simulink model "UAV_sync_unknown_sim"  (R2018b)
settings: Solver=ode23tb  StartTime=0.0  StopTime=35  RelTol=1e-3
values from neighbouring files (symbols this model uses):
  Bm = [zeros(6,6); eye(6)]    [UAV_sync_unknown.m]    (also in UAV_sync_unknown_gap.m)
  C_rho = 1.225    [SC42120_UAV_Preconditions.m]
  D0 = [M0 0 0 0 0 0 ... (first row only)    [SC42120_UAV_Preconditions.m]
  Derivative_gain_phi = 50    [SC42120_UAV_Preconditions.m]
  Derivative_gain_psi = 50    [SC42120_UAV_Preconditions.m]
  Derivative_gain_theta = 50    [SC42120_UAV_Preconditions.m]
  Derivative_gain_x = 50    [SC42120_UAV_Preconditions.m]
  Derivative_gain_y = 50    [SC42120_UAV_Preconditions.m]
  Derivative_gain_z = 50    [SC42120_UAV_Preconditions.m]
  G = 9.80665    [SC42120_UAV_Preconditions.m]
  g0 = [0;0;-M0*G;0;0;0]    [SC42120_UAV_Preconditions.m]
  I0 = [0.02 0 -0.01 ... (first row only)    [SC42120_UAV_Preconditions.m]
  InitWind = [0;0;0]    [SC42120_UAV_Preconditions.m]
  Kp = diag(P)    [SC42120_UAV_Preconditions.m]
  Kv = diag(V)    [SC42120_UAV_Preconditions.m]
  M0 = 10    [SC42120_UAV_Preconditions.m]
  M1 = 20    [UAV_sync_known.m]    (also in UAV_sync_unknown.m; UAV_sync_unknown_gap.m)
  M2 = 30    [UAV_sync_known.m]    (also in UAV_sync_unknown.m; UAV_sync_unknown_gap.m)
  M3 = 40    [UAV_sync_known.m]    (also in UAV_sync_unknown.m; UAV_sync_unknown_gap.m)
  M4 = 50    [UAV_sync_known.m]    (also in UAV_sync_unknown.m; UAV_sync_unknown_gap.m)
  P = [Proportional_x Proportional_y Proportional_z Proportional_phi Proportional_theta Proportional_psi]    [SC42120_UAV_Preconditions.m]    (also in UAV_sync_unknown.m = lyap(Am',Q); UAV_sync_unknown_gap.m = lyap(Am',Q); drawDATCOMaircraft.m = temparray)
  Proportional_phi = 50    [SC42120_UAV_Preconditions.m]
  Proportional_psi = 50    [SC42120_UAV_Preconditions.m]
  Proportional_theta = 50    [SC42120_UAV_Preconditions.m]
  Proportional_x = 50    [SC42120_UAV_Preconditions.m]
  Proportional_y = 50    [SC42120_UAV_Preconditions.m]
  Proportional_z = 50    [SC42120_UAV_Preconditions.m]
undefined symbols (not defined in the file or in its folder): Aero, APlane, Bxl, C, Ctr, deg, DiscIntNeverNeededParam, F, Guid, Init, Light, MIL, Path, rad, s, Trim, Utility
libraries: aerolibconvert2 x37, sharedutil x18, simulink x15, dspsigops x7, shared6dof x6, aerolibasang x4, simulink_extras x3, aerolibadyn x1, aerolibtransform2 x1, aerolibwind2 x1
(part 2 of 7)

== system UAV_sync_unknown_sim/Node 0/VF Approach/ENVIRONMENT ==
  note: Wind slowly time varying
  note: Dynamic wind
  note: Constant wind
  PlantData : Inport
  Bus Creator : BusCreator  Inputs=4
  Bus Selector1 : BusSelector  OutputSignals=xyh,Velocity (inertial),From inertial to body matrix
  Bus Selector2 : BusSelector  OutputSignals=From inertial to body matrix
  Bus Selector3 : BusSelector  OutputSignals=PlantData
  Bus Selector4 : BusSelector  OutputSignals=From inertial to body matrix
  Constant1 : Constant  Value=Init.windConst
  Dot Product : DotProduct  InputSameDT=on  OutDataTypeStr=Inherit: Inherit via internal rule
  Dryden Wind Turbulence Model (Continuous (+q +r)) : aerolibwind2/Dryden Wind Turbulence Model  (Continuous (+q -r))  units=Metric (MKS)  spec=MIL-F-8785C  model=Continuous Dryden (+q +r)  W20=10  Wdeg=135  TurbProb=10^-2 - Light  L_high=533.4  Wingspan=Bxl.b  ts=0.1  Seed=[23341 23342 23343 23344]  T_on=on
      settings: SourceProductName=Aerospace Blockset
  Height : Selector  InputPortWidth=3  IndexOptions=Index vector (dialog)  Indices=3  OutputSizes=1
  Init.DryOnOff : Gain  Gain=Init.DryOnOff
  "Init.DryOnOff " : Gain  Gain=Init.DryOnOff
  Init.WTimevar : Gain  Gain=Init.WTimevar
  Product : Product  Multiplication=Matrix(*)
  "Product " : Product  Multiplication=Matrix(*)
  Slowly time varying wind gen. : Subsystem
  Sum1 : Sum  Inputs=|++
  Sum3 : Sum  Inputs=|++
  Vt : Sqrt  SaturateOnIntegerOverflow=on
  EnvData : Outport
  wires:
  Bus Selector1/1 -> Height/1  "<xyh>"
  Bus Selector1/2 -> Dot Product/2, Dot Product/1  "<Velocity (inertial)>"
  Bus Selector1/3 -> Dryden Wind Turbulence Model (Continuous (+q +r))/3  "<From inertial to body matrix>"
  Bus Selector3/1 -> Bus Selector4/1, Bus Selector1/1, Bus Selector2/1  "<PlantData>"
  Height/1 -> Dryden Wind Turbulence Model (Continuous (+q +r))/1  "Altitude"
  Dot Product/1 -> Vt/1
  Vt/1 -> Dryden Wind Turbulence Model (Continuous (+q +r))/2  "Speed"
  Sum1/1 -> Bus Creator/3, Sum3/2  "Wind velocity (dyn) (body)"
  Constant1/1 -> Product/2
  Bus Creator/1 -> EnvData/1
  "Init.DryOnOff "/1 -> Bus Creator/4  "Wind ang rate (dyn) (body)"
  Sum3/1 -> Bus Creator/2  "Wind total (body)"
  Dryden Wind Turbulence Model (Continuous (+q +r))/1 -> Init.DryOnOff/1
  Bus Selector2/1 -> Product/1  "<From inertial to body matrix>"
  Dryden Wind Turbulence Model (Continuous (+q +r))/2 -> "Init.DryOnOff "/1
  PlantData/1 -> Bus Selector3/1
  Product/1 -> Bus Creator/1, Sum3/1  "Wind velocity (sta) (body)"
  Bus Selector4/1 -> "Product "/1  "<From inertial to body matrix>"
  Init.WTimevar/1 -> Sum1/2  "Wind slowly time varying"
  Init.DryOnOff/1 -> Sum1/1
  "Product "/1 -> Init.WTimevar/1
  Slowly time varying wind gen./1(Out1) -> "Product "/2

== system UAV_sync_unknown_sim/Node 0/VF Approach/GROUND HIT ==
  PlantData : Inport
  Bus Selector1 : BusSelector  OutputSignals=xyh
  Bus Selector3 : BusSelector  OutputSignals=PlantData
  Constant : Constant  Value=0
  Relational Operator : RelationalOperator  Operator=<=  OutDataTypeStr=boolean  RndMeth=Simplest
  Selector : Selector  InputPortWidth=3  IndexOptions=Index vector (dialog)  Indices=3  OutputSizes=1
  Stop Simulation : Stop
  wires:
  PlantData/1 -> Bus Selector3/1
  Selector/1 -> Relational Operator/1
  Bus Selector1/1 -> Selector/1  "<xyh>"
  Constant/1 -> Relational Operator/2
  Relational Operator/1 -> Stop Simulation/1
  Bus Selector3/1 -> Bus Selector1/1  "<PlantData>"

== system UAV_sync_unknown_sim/Node 0/VF Approach/MANUAL INPUTS ==
  note: Manual control
      |
      | The switches below enable (up position) or disable (down position) the manual control in the Visual Interface sub-block.
      | (default: down)
  note: Open-loop inputs
      |
      | The switches below enables a custom input from the Workspace (timeseries data type) to the control surfaces.
  note: Trim condition
      |
      | The sub-block below allows to try the actuators configuration for a trimmed flight.
  CtrBus : Inport
  EnvData : Inport  Port=2
  VF : Inport  Port=3
  GuidData : Inport  Port=4
  Bus Creator : BusCreator  Inputs=7
  Bus Selector : BusSelector  OutputSignals=throttle,ailerons,elevator,rudder
  Bus Selector1 : BusSelector  OutputSignals=Out_references,Target_height,Target_airspeed
  "CtrBus " : InportShadow
  From Workspace1 : FromWorkspace  Commented=on  VariableName=LogData.RCIN.ElevDem_IN  SampleTime=0.001
  From Workspace2 : FromWorkspace  Commented=on  VariableName=LogData.RCIN.RuddDem_IN  SampleTime=0.001
  From Workspace3 : FromWorkspace  Commented=on  VariableName=LogData.RCIN.ThrottleDem_IN  SampleTime=0.001
  From Workspace4 : FromWorkspace  Commented=on  VariableName=LogData.RCIN.AilDem_IN  SampleTime=0.001
  Goto4 : Goto  Commented=on  GotoTag=throttle
  Manual Switch{,1..7} (8 alike) : ManualSwitch  CurrentSetting=0
  Manual_cmd{,4..6} (4 alike) : Constant  Value=0
  Trim conditions : Subsystem
  CtrBus. : Outport
  EnvData. : Outport  Port=2
  GuidData. : Outport  Port=3
  VF. : Outport  Port=4
  wires:
  Manual Switch4/1 -> Goto4/1, Bus Creator/1  "throttle"
  Manual Switch7/1 -> Bus Creator/3  "elevator"
  Manual_cmd/1 -> Manual Switch/1
  Manual_cmd4/1 -> Manual Switch1/1
  Manual Switch5/1 -> Bus Creator/2  "ailerons"
  Manual Switch6/1 -> Bus Creator/4  "rudder"
  Manual_cmd6/1 -> Manual Switch3/1
  Manual_cmd5/1 -> Manual Switch2/1
  Bus Creator/1 -> CtrBus./1
  Manual Switch1/1 -> Manual Switch5/2  "ailerons"
  Manual Switch2/1 -> Manual Switch7/2  "elevator"
  Manual Switch3/1 -> Manual Switch6/2  "rudder"
  From Workspace3/1 -> Manual Switch4/1
  Manual Switch/1 -> Manual Switch4/2
  Bus Selector/1 -> Trim conditions/1(throttle)  "<throttle>"
  Trim conditions/1(throttout) -> Manual Switch/2
  Bus Selector/2 -> Trim conditions/2(ail)  "<ailerons>"
  Bus Selector/3 -> Trim conditions/3(elev)  "<elevator>"
  Bus Selector/4 -> Trim conditions/4(rudd)  "<rudder>"
  Trim conditions/4(ruddout) -> Manual Switch3/2
  Trim conditions/2(ailout) -> Manual Switch1/2
  Trim conditions/3(elevout) -> Manual Switch2/2
  EnvData/1 -> EnvData./1
  From Workspace4/1 -> Manual Switch5/1
  From Workspace1/1 -> Manual Switch7/1
  From Workspace2/1 -> Manual Switch6/1
  GuidData/1 -> GuidData./1
  VF/1 -> VF./1
  CtrBus/1 -> Bus Selector/1
  "CtrBus "/1 -> Bus Selector1/1
  Bus Selector1/1 -> Bus Creator/5  "<Out_references>"
  Bus Selector1/2 -> Bus Creator/6  "<Target_height>"
  Bus Selector1/3 -> Bus Creator/7  "<Target_airspeed>"

== system UAV_sync_unknown_sim/Node 0/VF Approach/PATH FOLLOWING ==
  note: Out
  note: Ground speed(s) calculation
  note: Output merge
  note: Path following
      |
      | Each subsystem is enabled by the 'flag' variable according to the path manager choice or user configuration.
      | If you want to use only the path following for a single line/orbit simulation, then disable the Path manager.
      |
      | GPS-derived signals, such as the inertial position and the course angle use a 10 Hz sampling time to reflect real signal on-board acquisition.
  PlantData : Inport
  DerCond : Inport  Port=2
  EnvData : Inport  Port=3
  GuidData : Inport  Port=4
  Angle Conversion : aerolibconvert2/Angle Conversion  IU=rad  OU=deg
  Bus Creator : BusCreator  Inputs=7
  Bus Selector{1,4,6,8} (4 alike) : BusSelector  OutputSignals=PlantData
  Bus Selector2 : BusSelector  OutputSignals=DerCond
  Bus Selector3 : BusSelector  OutputSignals=DerCond
  Bus Selector5 : BusSelector  OutputSignals=Path flag
  Constant6 : Constant  Value=0
  Data Type Conversion : DataTypeConversion  OutDataTypeStr=boolean
  "DerCond " : InportShadow  Port=2
  "EnvData " : InportShadow  Port=3
  Extract Vg : Subsystem
  Extract Vg_prime : Subsystem
  "GuidData " : InportShadow  Port=4
  Logical Operator : Logic  Operator=NOT  AllPortsSameDT=off  OutDataTypeStr=boolean
  Manual Switch1 : ManualSwitch  CurrentSetting=0
  Merge{,1..3} (4 alike) : Merge
  Orbit Path Following (Enabled Subsystem) : Subsystem  TreatAsAtomicUnit=on
  "PlantData " : InportShadow
  "PlantData  " : InportShadow
  "PlantData   " : InportShadow
  Scope : Scope
  Straight-line Path Following (Enabled Subsystem) : Subsystem  TreatAsAtomicUnit=on
  "PlantData. " : Outport
  "DerCond. " : Outport  Port=2
  EnvData. : Outport  Port=3
  VF. : Outport  Port=4
  GuidData. : Outport  Port=5
  wires:
  Merge/1 -> Manual Switch1/2
  Constant6/1 -> Manual Switch1/1
  EnvData/1 -> EnvData./1
  PlantData/1 -> Bus Selector4/1, Bus Selector1/1
  Bus Selector1/1 -> Straight-line Path Following (Enabled Subsystem)/1(PlantData)  "<PlantData>"
  DerCond/1 -> Bus Selector2/1, Bus Selector3/1
  Bus Creator/1 -> VF./1
  Manual Switch1/1 -> Bus Creator/2, Angle Conversion/1  "chi_c"
  Logical Operator/1 -> Orbit Path Following (Enabled Subsystem)/Enable
  Bus Selector4/1 -> Orbit Path Following (Enabled Subsystem)/1(PlantData)  "<PlantData>"
  Bus Selector3/1 -> Orbit Path Following (Enabled Subsystem)/2(DerCond)  "<DerCond>"
  Data Type Conversion/1 -> [path_flag], Straight-line Path Following (Enabled Subsystem)/Enable
  [path_flag] -> Logical Operator/1
  Bus Selector2/1 -> Straight-line Path Following (Enabled Subsystem)/2(DerCond)  "<DerCond>"
  Merge1/1 -> Bus Creator/3, Scope/1  "Vg_hat"
  [Vg_prime] -> Bus Creator/4  "Vg_prime"
  Straight-line Path Following (Enabled Subsystem)/2(Vg_hat_SL) -> [Vg_hat_SL]
  Straight-line Path Following (Enabled Subsystem)/3(chi_d_SL) -> [chi_d_SL]
  Straight-line Path Following (Enabled Subsystem)/4(chi_c_SL) -> [chi_c_SL]
  Orbit Path Following (Enabled Subsystem)/2(Vg_hat_O) -> [Vg_hat_O]
  Orbit Path Following (Enabled Subsystem)/3(chi_d_O) -> [chi_d_O]
  Orbit Path Following (Enabled Subsystem)/1(chi_c_O) -> [chi_c_O]
  [chi_c_SL] -> Merge/1
  [chi_c_O] -> Merge/2
  [Vg_hat_O] -> Merge1/2
  [Vg_hat_SL] -> Merge1/1
  [chi_d_O] -> Merge2/2
  [chi_d_SL] -> Merge2/1
  Merge2/1 -> Bus Creator/6  "chi_d"
  Angle Conversion/1 -> Bus Creator/1  "chi_c_deg"
  Straight-line Path Following (Enabled Subsystem)/1(e_y) -> [e_y]
  [e_y] -> Merge3/1
  Orbit Path Following (Enabled Subsystem)/4(d_tilde) -> [d_tilde]
  [d_tilde] -> Merge3/2
  Merge3/1 -> Bus Creator/7  "xtrack_erorr"
  GuidData/1 -> Bus Selector5/1, Orbit Path Following (Enabled Subsystem)/3(GuidData), Straight-line Path Following (Enabled Subsystem)/3(GuidData)
  Bus Selector5/1 -> Data Type Conversion/1  "<Path flag>"
  "DerCond "/1 -> "DerCond. "/1
  "GuidData "/1 -> GuidData./1
  "PlantData "/1 -> "PlantData. "/1
  Extract Vg_prime/1(Vg') -> [Vg_prime]
  Bus Selector6/1 -> Extract Vg_prime/1(PlantData)  "<PlantData>"
  [V_g] -> Bus Creator/5  "V_g"
  Extract Vg/1(Vg) -> [V_g]
  "PlantData  "/1 -> Bus Selector6/1
  [V_g] -> Straight-line Path Following (Enabled Subsystem)/4(Vg)
  [V_g] -> Orbit Path Following (Enabled Subsystem)/4(Vg)
  [Vg_prime] -> Straight-line Path Following (Enabled Subsystem)/5(Vg_prime)
  [Vg_prime] -> Orbit Path Following (Enabled Subsystem)/5(Vg_prime)
  "EnvData "/1 -> Extract Vg/2(EnvData)
  "PlantData   "/1 -> Bus Selector8/1
  Bus Selector8/1 -> Extract Vg/1(PlantData)  "<PlantData>"

== system UAV_sync_unknown_sim/Node 0/VF Approach/PATH MANAGER ==
  note: Path following only
  note: Path manager
  PlantData : Inport
  DerCond : Inport  Port=2
  EnvData : Inport  Port=3
  Bus Selector : BusSelector  OutputSignals=PlantData.Position (inertial)
  Constant : Constant  Value=Path.onOff
  Constant1 : Constant  Value=Path.onOff
  Data Type Conversion : DataTypeConversion  OutDataTypeStr=boolean
  Enabled Subsystem : Subsystem  TreatAsAtomicUnit=on
  Fcn : Fcn  Commented=on  Expr=u(1)
  Fcn1 : Fcn  Commented=on  Expr=u(2)
  Logical Operator : Logic  Operator=NOT  AllPortsSameDT=off  OutDataTypeStr=boolean
  Merge : Merge
  Path Following data : Subsystem  TreatAsAtomicUnit=on
  XY Graph : simulink/Sinks/XY Graph  Commented=on  xmin=-50  xmax=600  ymin=-50  ymax=600  st=0.1
  Plantdata. : Outport
  DerCond. : Outport  Port=2
  EnvData. : Outport  Port=3
  GuidData. : Outport  Port=4
  wires:
  PlantData/1 -> Bus Selector/1, Plantdata./1
  DerCond/1 -> DerCond./1
  EnvData/1 -> EnvData./1
  Bus Selector/1 -> Fcn1/1, Fcn/1, Enabled Subsystem/1(xy)  "<Position (inertial)>"
  Merge/1 -> GuidData./1
  Constant/1 -> Data Type Conversion/1
  Data Type Conversion/1 -> Enabled Subsystem/Enable
  Constant1/1 -> Logical Operator/1
  Logical Operator/1 -> Path Following data/Enable
  Enabled Subsystem/1(GuidData) -> Merge/1
  Path Following data/1(GuidData) -> Merge/2
  Fcn/1 -> XY Graph/1
  Fcn1/1 -> XY Graph/2

== system UAV_sync_unknown_sim/Node 0/VF Approach/TO WORKSPACE ==
  PlantData : Inport
  DerCond : Inport  Port=2
  ControlBus : Inport  Port=3
  VF : Inport  Port=4
  GuidData : Inport  Port=5
  EnvData : Inport  Port=6
  Bus Creator : BusCreator  Inputs=6
  Bus Selector4 : BusSelector  OutputSignals=DerCond
  Bus Selector5 : BusSelector  OutputSignals=PlantData
  Sample at 0.01s : ZeroOrderHold  SampleTime=0.01
  To Workspace2 : ToWorkspace  VariableName=SimOut  SaveFormat=Timeseries  SampleTime=-1
      settings: Save2DSignal=2-D array (concatenate along first dimension)
  wires:
  Bus Creator/1 -> Sample at 0.01s/1
  Bus Selector5/1 -> Bus Creator/1  "<PlantData>"
  PlantData/1 -> Bus Selector5/1
  ControlBus/1 -> Bus Creator/3  "ControlBus"
  DerCond/1 -> Bus Selector4/1
  Bus Selector4/1 -> Bus Creator/2  "<DerCond>"
  GuidData/1 -> Bus Creator/5  "GuidData"
  VF/1 -> Bus Creator/4  "VF"
  EnvData/1 -> Bus Creator/6  "EnvData"
  Sample at 0.01s/1 -> To Workspace2/1

== system UAV_sync_unknown_sim/Node 1/Node 1/eps_c1_transpose ==
  euler angles : Inport
  Constant : Constant  Value=zeros(3)
  Constant1 : Constant  Value=zeros(6,1)
  Constant{2..3,6..7} (4 alike) : Constant  Value=0
  Constant4 : Constant  Value=zeros(3)
  Constant5 : Constant  Value=zeros(6,1)
  Constant8 : Constant  Value=zeros(3)
  Constant9 : Constant  Value=zeros(6,1)
  Create 3x3 Matrix{,1..3} (4 alike) : sharedutil/Create 3x3 Matrix  aMode=aMode
  Demux : Demux  Outputs=3
  Gain{,1..7} (8 alike) : Gain  Gain=-1
  Matrix Concatenate{,2,5..6} (4 alike) : Concatenate  Mode=Multidimensional array
  Matrix Concatenate{1,3..4,7..9} (6 alike) : Concatenate  Mode=Multidimensional array  ConcatenateDimension=2
  eps_c : Outport
  wires:
  euler angles/1 -> Demux/1
  Demux/1 -> Gain6/1, Create 3x3 Matrix3/2, Gain/1, Create 3x3 Matrix/6, Create 3x3 Matrix1/7, Gain3/1  "p"
  Gain/1 -> Create 3x3 Matrix/8
  Demux/2 -> Create 3x3 Matrix2/1, Gain4/1, Create 3x3 Matrix/7, Gain1/1  "q"
  Gain1/1 -> Create 3x3 Matrix/3
  Demux/3 -> Gain7/1, Create 3x3 Matrix3/6, Create 3x3 Matrix2/5, Gain5/1, Gain2/1, Create 3x3 Matrix/2  "r"
  Gain2/1 -> Create 3x3 Matrix/4
  Create 3x3 Matrix/1 -> Matrix Concatenate/1
  Constant/1 -> Matrix Concatenate/2
  Matrix Concatenate/1 -> Matrix Concatenate1/1
  Constant1/1 -> Matrix Concatenate1/2
  Constant2/1 -> Create 3x3 Matrix/9, Create 3x3 Matrix/5, Create 3x3 Matrix/1
  Constant3/1 -> Create 3x3 Matrix1/8, Create 3x3 Matrix1/6, Create 3x3 Matrix1/4, Create 3x3 Matrix1/3, Create 3x3 Matrix1/2, Create 3x3 Matrix1/1
  Gain3/1 -> Create 3x3 Matrix1/5
  Gain4/1 -> Create 3x3 Matrix1/9
  Create 3x3 Matrix1/1 -> Matrix Concatenate2/2
  Constant4/1 -> Matrix Concatenate2/1
  Matrix Concatenate1/1 -> Matrix Concatenate3/1
  Matrix Concatenate2/1 -> Matrix Concatenate3/2
  Matrix Concatenate3/1 -> Matrix Concatenate4/1
  Constant5/1 -> Matrix Concatenate4/2
  Gain5/1 -> Create 3x3 Matrix2/3
  Constant6/1 -> Create 3x3 Matrix2/9, Create 3x3 Matrix2/8, Create 3x3 Matrix2/7, Create 3x3 Matrix2/6, Create 3x3 Matrix2/4, Create 3x3 Matrix2/2
  Gain6/1 -> Create 3x3 Matrix3/4
  Gain7/1 -> Create 3x3 Matrix3/8
  Constant7/1 -> Create 3x3 Matrix3/9, Create 3x3 Matrix3/7, Create 3x3 Matrix3/5, Create 3x3 Matrix3/3, Create 3x3 Matrix3/1
  Create 3x3 Matrix2/1 -> Matrix Concatenate5/2
  Constant8/1 -> Matrix Concatenate6/1, Matrix Concatenate5/1
  Create 3x3 Matrix3/1 -> Matrix Concatenate6/2
  Constant9/1 -> Matrix Concatenate7/2
  Matrix Concatenate5/1 -> Matrix Concatenate7/1
  Matrix Concatenate7/1 -> Matrix Concatenate8/1
  Matrix Concatenate6/1 -> Matrix Concatenate8/2
  Matrix Concatenate4/1 -> Matrix Concatenate9/1
  Matrix Concatenate8/1 -> Matrix Concatenate9/2
  Matrix Concatenate9/1 -> eps_c/1

== system UAV_sync_unknown_sim/Node 1/Node 1/eps_g ==
  euler angles : Inport
  Cos : Trigonometry  Operator=cos
  Cos1 : Trigonometry  Operator=cos
  Demux : Demux  Outputs=3
  Gain : Gain  Gain=G
  Gain1 : Gain  Gain=G
  Gain2 : Gain  Gain=G
  Gain3 : Gain  Gain=-1
  Gain4 : Gain  Gain=-1
  Multiply : Product
  Multiply1 : Product
  Mux : Mux  Inputs=6
  Sin : Trigonometry
  Sin1 : Trigonometry
  Sin2 : Trigonometry  Operator=cos
  Terminator : Terminator
  Zero : Constant  Value=0  OutDataTypeStr=Inherit: Inherit via back propagation
  eps_g : Outport
  wires:
  euler angles/1 -> Demux/1
  Sin/1 -> Gain/1
  Cos/1 -> Multiply/1
  Sin1/1 -> Multiply/2
  Multiply/1 -> Gain1/1
  Cos1/1 -> Multiply1/1
  Sin2/1 -> Multiply1/2
  Multiply1/1 -> Gain2/1
  Gain/1 -> Mux/1
  Gain1/1 -> Gain3/1
  Gain2/1 -> Gain4/1
  Zero/1 -> Mux/6, Mux/4, Mux/5
  Mux/1 -> eps_g/1
  Gain3/1 -> Mux/2
  Gain4/1 -> Mux/3
  Demux/1 -> Cos1/1, Sin1/1
  Demux/2 -> Sin2/1, Cos/1, Sin/1
  Demux/3 -> Terminator/1

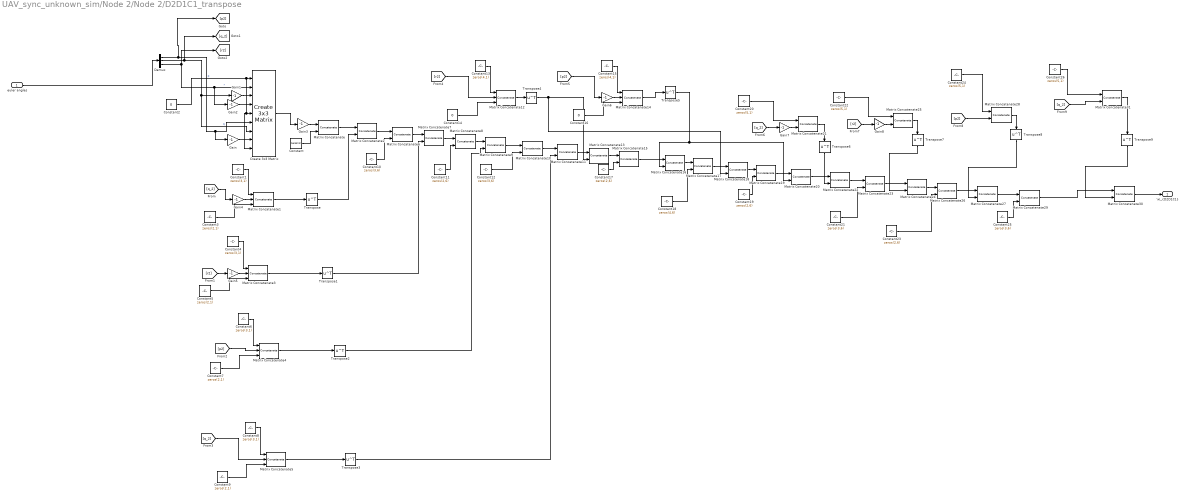
== system UAV_sync_unknown_sim/Node 2/Node 2/D2D1C1_transpose ==
  euler angles : Inport
  Constant : Constant  Value=zeros(3)
  Constant{1,4,6,8} (4 alike) : Constant  Value=zeros(3,1)
  Constant{10,12,21,25} (4 alike) : Constant  Value=zeros(3,6)
  Constant{11,17,19,23} (4 alike) : Constant  Value=zeros(2,6)
  Constant13 : Constant  Value=zeros(4,1)
  Constant14 : Constant  Value=0
  Constant15 : Constant  Value=zeros(4,1)
  Constant16 : Constant  Value=0
  Constant18 : Constant  Value=zeros(4,6)
  Constant2 : Constant  Value=0
  Constant{20,22,24,26} (4 alike) : Constant  Value=zeros(5,1)
  Constant{3,5,7,9} (4 alike) : Constant  Value=zeros(2,1)
  Create 3x3 Matrix : sharedutil/Create 3x3 Matrix  aMode=aMode
  Demux : Demux  Outputs=3
  Gain{,1..8} (9 alike) : Gain  Gain=-1
  Matrix Concatenate : Concatenate  Mode=Multidimensional array  ConcatenateDimension=2
  Matrix Concatenate{1,3..5,12,14} (6 alike) : Concatenate  NumInputs=3  Mode=Multidimensional array
  Matrix Concatenate{2,6..11,13,15..31} (25 alike) : Concatenate  Mode=Multidimensional array
  Transpose{,1..9} (10 alike) : Math  Operator=transpose  SaturateOnIntegerOverflow=on
  "\\xi_{D2D1C1}" : Outport
  wires:
  euler angles/1 -> Demux/1
  Demux/1 -> [p2], Gain/1, Create 3x3 Matrix/6  "p"
  Gain/1 -> Create 3x3 Matrix/8
  Demux/2 -> [q_2], Create 3x3 Matrix/7, Gain1/1  "q"
  Gain1/1 -> Create 3x3 Matrix/3
  Demux/3 -> Gain2/1, Create 3x3 Matrix/2, [r2]  "r"
  Gain2/1 -> Create 3x3 Matrix/4
  Create 3x3 Matrix/1 -> Gain3/1
  Constant/1 -> Matrix Concatenate/2
  Matrix Concatenate/1 -> Matrix Concatenate2/1
  Constant2/1 -> Create 3x3 Matrix/9, Create 3x3 Matrix/5, Create 3x3 Matrix/1
  Gain3/1 -> Matrix Concatenate/1
  Constant1/1 -> Matrix Concatenate1/1
  Constant3/1 -> Matrix Concatenate1/3
  Gain4/1 -> Matrix Concatenate1/2
  Matrix Concatenate1/1 -> Transpose/1
  Gain5/1 -> Matrix Concatenate3/2
  Constant5/1 -> Matrix Concatenate3/3
  Constant4/1 -> Matrix Concatenate3/1
  Constant7/1 -> Matrix Concatenate4/3
  Constant6/1 -> Matrix Concatenate4/1
  Constant9/1 -> Matrix Concatenate5/3
  Constant8/1 -> Matrix Concatenate5/1
  [q_2] -> Gain4/1
  [r2] -> Gain5/1
  [p2] -> Matrix Concatenate4/2
  [q_2] -> Matrix Concatenate5/2
  Matrix Concatenate2/1 -> Matrix Concatenate6/1
  Constant10/1 -> Matrix Concatenate6/2
  Matrix Concatenate6/1 -> Matrix Concatenate7/1
  Matrix Concatenate3/1 -> Transpose1/1
  Matrix Concatenate7/1 -> Matrix Concatenate8/1
  Matrix Concatenate8/1 -> Matrix Concatenate9/1
  Constant11/1 -> Matrix Concatenate8/2
  Matrix Concatenate4/1 -> Transpose2/1
  Matrix Concatenate9/1 -> Matrix Concatenate10/1
  Constant12/1 -> Matrix Concatenate10/2
  Matrix Concatenate10/1 -> Matrix Concatenate11/1
  Matrix Concatenate5/1 -> Transpose3/1
  Constant13/1 -> Matrix Concatenate12/1
  Constant14/1 -> Matrix Concatenate12/3
  [r2] -> Matrix Concatenate12/2
  Matrix Concatenate12/1 -> Transpose4/1
  Matrix Concatenate11/1 -> Matrix Concatenate13/1
  Constant16/1 -> Matrix Concatenate14/3
  [p2] -> Gain6/1
  Constant15/1 -> Matrix Concatenate14/1
  Gain6/1 -> Matrix Concatenate14/2
  Matrix Concatenate13/1 -> Matrix Concatenate15/1
  Constant17/1 -> Matrix Concatenate15/2
  Matrix Concatenate15/1 -> Matrix Concatenate16/1
  Matrix Concatenate14/1 -> Transpose5/1
  Matrix Concatenate16/1 -> Matrix Concatenate17/1
  Constant18/1 -> Matrix Concatenate17/2
  Matrix Concatenate17/1 -> Matrix Concatenate18/1
  Matrix Concatenate18/1 -> Matrix Concatenate19/1
  Constant19/1 -> Matrix Concatenate19/2
  Matrix Concatenate19/1 -> Matrix Concatenate20/1
  Constant20/1 -> Matrix Concatenate21/1
  Gain7/1 -> Matrix Concatenate21/2
  [q_2] -> Gain7/1
  Matrix Concatenate21/1 -> Transpose6/1
  Matrix Concatenate20/1 -> Matrix Concatenate22/1
  Matrix Concatenate22/1 -> Matrix Concatenate23/1
  Constant21/1 -> Matrix Concatenate23/2
  Matrix Concatenate23/1 -> Matrix Concatenate24/1
  Gain8/1 -> Matrix Concatenate25/2
  Constant22/1 -> Matrix Concatenate25/1
  [r2] -> Gain8/1
  Matrix Concatenate25/1 -> Transpose7/1
  Matrix Concatenate24/1 -> Matrix Concatenate26/1
  Constant23/1 -> Matrix Concatenate26/2
  Matrix Concatenate26/1 -> Matrix Concatenate27/1
  Matrix Concatenate28/1 -> Transpose8/1
  [p2] -> Matrix Concatenate28/2
  Constant24/1 -> Matrix Concatenate28/1
  Matrix Concatenate27/1 -> Matrix Concatenate29/1
  Constant25/1 -> Matrix Concatenate29/2
  Matrix Concatenate29/1 -> Matrix Concatenate30/1
  Constant26/1 -> Matrix Concatenate31/1
  [q_2] -> Matrix Concatenate31/2
  Matrix Concatenate31/1 -> Transpose9/1
  Matrix Concatenate30/1 -> "\\xi_{D2D1C1}"/1
  Transpose/1 -> Matrix Concatenate2/2
  Transpose1/1 -> Matrix Concatenate7/2
  Transpose2/1 -> Matrix Concatenate9/2
  Transpose3/1 -> Matrix Concatenate11/2
  Transpose4/1 -> Matrix Concatenate18/2, Matrix Concatenate13/2
  Transpose5/1 -> Matrix Concatenate16/2, Matrix Concatenate20/2
  Transpose6/1 -> Matrix Concatenate22/2
  Transpose7/1 -> Matrix Concatenate24/2
  Transpose8/1 -> Matrix Concatenate27/2
  Transpose9/1 -> Matrix Concatenate30/2

== system UAV_sync_unknown_sim/Node 2/Node 2/eps_c1_transpose ==
  euler angles : Inport
  Constant : Constant  Value=zeros(3)
  Constant1 : Constant  Value=zeros(6,1)
  Constant{2..3,6..7} (4 alike) : Constant  Value=0
  Constant4 : Constant  Value=zeros(3)
  Constant5 : Constant  Value=zeros(6,1)
  Constant8 : Constant  Value=zeros(3)
  Constant9 : Constant  Value=zeros(6,1)
  Create 3x3 Matrix{,1..3} (4 alike) : sharedutil/Create 3x3 Matrix  aMode=aMode
  Demux : Demux  Outputs=3
  Gain{,1..7} (8 alike) : Gain  Gain=-1
  Matrix Concatenate{,2,5..6} (4 alike) : Concatenate  Mode=Multidimensional array
  Matrix Concatenate{1,3..4,7..9} (6 alike) : Concatenate  Mode=Multidimensional array  ConcatenateDimension=2
  eps_c : Outport
  wires:
  euler angles/1 -> Demux/1
  Demux/1 -> Gain6/1, Create 3x3 Matrix3/2, Gain/1, Create 3x3 Matrix/6, Create 3x3 Matrix1/7, Gain3/1  "p"
  Gain/1 -> Create 3x3 Matrix/8
  Demux/2 -> Create 3x3 Matrix2/1, Gain4/1, Create 3x3 Matrix/7, Gain1/1  "q"
  Gain1/1 -> Create 3x3 Matrix/3
  Demux/3 -> Gain7/1, Create 3x3 Matrix3/6, Create 3x3 Matrix2/5, Gain5/1, Gain2/1, Create 3x3 Matrix/2  "r"
  Gain2/1 -> Create 3x3 Matrix/4
  Create 3x3 Matrix/1 -> Matrix Concatenate/1
  Constant/1 -> Matrix Concatenate/2
  Matrix Concatenate/1 -> Matrix Concatenate1/1
  Constant1/1 -> Matrix Concatenate1/2
  Constant2/1 -> Create 3x3 Matrix/9, Create 3x3 Matrix/5, Create 3x3 Matrix/1
  Constant3/1 -> Create 3x3 Matrix1/8, Create 3x3 Matrix1/6, Create 3x3 Matrix1/4, Create 3x3 Matrix1/3, Create 3x3 Matrix1/2, Create 3x3 Matrix1/1
  Gain3/1 -> Create 3x3 Matrix1/5
  Gain4/1 -> Create 3x3 Matrix1/9
  Create 3x3 Matrix1/1 -> Matrix Concatenate2/2
  Constant4/1 -> Matrix Concatenate2/1
  Matrix Concatenate1/1 -> Matrix Concatenate3/1
  Matrix Concatenate2/1 -> Matrix Concatenate3/2
  Matrix Concatenate3/1 -> Matrix Concatenate4/1
  Constant5/1 -> Matrix Concatenate4/2
  Gain5/1 -> Create 3x3 Matrix2/3
  Constant6/1 -> Create 3x3 Matrix2/9, Create 3x3 Matrix2/8, Create 3x3 Matrix2/7, Create 3x3 Matrix2/6, Create 3x3 Matrix2/4, Create 3x3 Matrix2/2
  Gain6/1 -> Create 3x3 Matrix3/4
  Gain7/1 -> Create 3x3 Matrix3/8
  Constant7/1 -> Create 3x3 Matrix3/9, Create 3x3 Matrix3/7, Create 3x3 Matrix3/5, Create 3x3 Matrix3/3, Create 3x3 Matrix3/1
  Create 3x3 Matrix2/1 -> Matrix Concatenate5/2
  Constant8/1 -> Matrix Concatenate6/1, Matrix Concatenate5/1
  Create 3x3 Matrix3/1 -> Matrix Concatenate6/2
  Constant9/1 -> Matrix Concatenate7/2
  Matrix Concatenate5/1 -> Matrix Concatenate7/1
  Matrix Concatenate7/1 -> Matrix Concatenate8/1
  Matrix Concatenate6/1 -> Matrix Concatenate8/2
  Matrix Concatenate4/1 -> Matrix Concatenate9/1
  Matrix Concatenate8/1 -> Matrix Concatenate9/2
  Matrix Concatenate9/1 -> eps_c/1

== system UAV_sync_unknown_sim/Node 2/Node 2/eps_g ==
  euler angles : Inport
  Cos : Trigonometry  Operator=cos
  Cos1 : Trigonometry  Operator=cos
  Demux : Demux  Outputs=3
  Gain : Gain  Gain=G
  Gain1 : Gain  Gain=G
  Gain2 : Gain  Gain=G
  Gain3 : Gain  Gain=-1
  Gain4 : Gain  Gain=-1
  Multiply : Product
  Multiply1 : Product
  Mux : Mux  Inputs=6
  Sin : Trigonometry
  Sin1 : Trigonometry
  Sin2 : Trigonometry  Operator=cos
  Terminator : Terminator
  Zero : Constant  Value=0  OutDataTypeStr=Inherit: Inherit via back propagation
  eps_g : Outport
  wires:
  euler angles/1 -> Demux/1
  Sin/1 -> Gain/1
  Cos/1 -> Multiply/1
  Sin1/1 -> Multiply/2
  Multiply/1 -> Gain1/1
  Cos1/1 -> Multiply1/1
  Sin2/1 -> Multiply1/2
  Multiply1/1 -> Gain2/1
  Gain/1 -> Mux/1
  Gain1/1 -> Gain3/1
  Gain2/1 -> Gain4/1
  Zero/1 -> Mux/6, Mux/4, Mux/5
  Mux/1 -> eps_g/1
  Gain3/1 -> Mux/2
  Gain4/1 -> Mux/3
  Demux/1 -> Cos1/1, Sin1/1
  Demux/2 -> Sin2/1, Cos/1, Sin/1
  Demux/3 -> Terminator/1

== system UAV_sync_unknown_sim/Node 3/Node 1/eps_c1_transpose ==
  euler angles : Inport
  Constant : Constant  Value=zeros(3)
  Constant1 : Constant  Value=zeros(6,1)
  Constant{2..3,6..7} (4 alike) : Constant  Value=0
  Constant4 : Constant  Value=zeros(3)
  Constant5 : Constant  Value=zeros(6,1)
  Constant8 : Constant  Value=zeros(3)
  Constant9 : Constant  Value=zeros(6,1)
  Create 3x3 Matrix{,1..3} (4 alike) : sharedutil/Create 3x3 Matrix  aMode=aMode
  Demux : Demux  Outputs=3
  Gain{,1..7} (8 alike) : Gain  Gain=-1
  Matrix Concatenate{,2,5..6} (4 alike) : Concatenate  Mode=Multidimensional array
  Matrix Concatenate{1,3..4,7..9} (6 alike) : Concatenate  Mode=Multidimensional array  ConcatenateDimension=2
  eps_c : Outport
  wires:
  euler angles/1 -> Demux/1
  Demux/1 -> Gain6/1, Create 3x3 Matrix3/2, Gain/1, Create 3x3 Matrix/6, Create 3x3 Matrix1/7, Gain3/1  "p"
  Gain/1 -> Create 3x3 Matrix/8
  Demux/2 -> Create 3x3 Matrix2/1, Gain4/1, Create 3x3 Matrix/7, Gain1/1  "q"
  Gain1/1 -> Create 3x3 Matrix/3
  Demux/3 -> Gain7/1, Create 3x3 Matrix3/6, Create 3x3 Matrix2/5, Gain5/1, Gain2/1, Create 3x3 Matrix/2  "r"
  Gain2/1 -> Create 3x3 Matrix/4
  Create 3x3 Matrix/1 -> Matrix Concatenate/1
  Constant/1 -> Matrix Concatenate/2
  Matrix Concatenate/1 -> Matrix Concatenate1/1
  Constant1/1 -> Matrix Concatenate1/2
  Constant2/1 -> Create 3x3 Matrix/9, Create 3x3 Matrix/5, Create 3x3 Matrix/1
  Constant3/1 -> Create 3x3 Matrix1/8, Create 3x3 Matrix1/6, Create 3x3 Matrix1/4, Create 3x3 Matrix1/3, Create 3x3 Matrix1/2, Create 3x3 Matrix1/1
  Gain3/1 -> Create 3x3 Matrix1/5
  Gain4/1 -> Create 3x3 Matrix1/9
  Create 3x3 Matrix1/1 -> Matrix Concatenate2/2
  Constant4/1 -> Matrix Concatenate2/1
  Matrix Concatenate1/1 -> Matrix Concatenate3/1
  Matrix Concatenate2/1 -> Matrix Concatenate3/2
  Matrix Concatenate3/1 -> Matrix Concatenate4/1
  Constant5/1 -> Matrix Concatenate4/2
  Gain5/1 -> Create 3x3 Matrix2/3
  Constant6/1 -> Create 3x3 Matrix2/9, Create 3x3 Matrix2/8, Create 3x3 Matrix2/7, Create 3x3 Matrix2/6, Create 3x3 Matrix2/4, Create 3x3 Matrix2/2
  Gain6/1 -> Create 3x3 Matrix3/4
  Gain7/1 -> Create 3x3 Matrix3/8
  Constant7/1 -> Create 3x3 Matrix3/9, Create 3x3 Matrix3/7, Create 3x3 Matrix3/5, Create 3x3 Matrix3/3, Create 3x3 Matrix3/1
  Create 3x3 Matrix2/1 -> Matrix Concatenate5/2
  Constant8/1 -> Matrix Concatenate6/1, Matrix Concatenate5/1
  Create 3x3 Matrix3/1 -> Matrix Concatenate6/2
  Constant9/1 -> Matrix Concatenate7/2
  Matrix Concatenate5/1 -> Matrix Concatenate7/1
  Matrix Concatenate7/1 -> Matrix Concatenate8/1
  Matrix Concatenate6/1 -> Matrix Concatenate8/2
  Matrix Concatenate4/1 -> Matrix Concatenate9/1
  Matrix Concatenate8/1 -> Matrix Concatenate9/2
  Matrix Concatenate9/1 -> eps_c/1

== system UAV_sync_unknown_sim/Node 3/Node 1/eps_g ==
  euler angles : Inport
  Cos : Trigonometry  Operator=cos
  Cos1 : Trigonometry  Operator=cos
  Demux : Demux  Outputs=3
  Gain : Gain  Gain=G
  Gain1 : Gain  Gain=G
  Gain2 : Gain  Gain=G
  Gain3 : Gain  Gain=-1
  Gain4 : Gain  Gain=-1
  Multiply : Product
  Multiply1 : Product
  Mux : Mux  Inputs=6
  Sin : Trigonometry
  Sin1 : Trigonometry
  Sin2 : Trigonometry  Operator=cos
  Terminator : Terminator
  Zero : Constant  Value=0  OutDataTypeStr=Inherit: Inherit via back propagation
  eps_g : Outport
  wires:
  euler angles/1 -> Demux/1
  Sin/1 -> Gain/1
  Cos/1 -> Multiply/1
  Sin1/1 -> Multiply/2
  Multiply/1 -> Gain1/1
  Cos1/1 -> Multiply1/1
  Sin2/1 -> Multiply1/2
  Multiply1/1 -> Gain2/1
  Gain/1 -> Mux/1
  Gain1/1 -> Gain3/1
  Gain2/1 -> Gain4/1
  Zero/1 -> Mux/6, Mux/4, Mux/5
  Mux/1 -> eps_g/1
  Gain3/1 -> Mux/2
  Gain4/1 -> Mux/3
  Demux/1 -> Cos1/1, Sin1/1
  Demux/2 -> Sin2/1, Cos/1, Sin/1
  Demux/3 -> Terminator/1

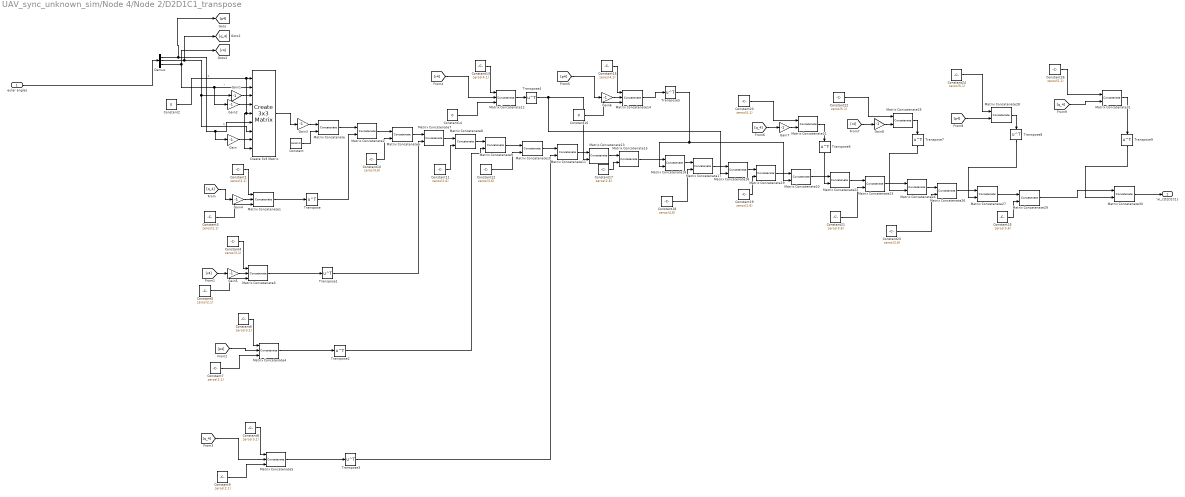
== system UAV_sync_unknown_sim/Node 4/Node 2/D2D1C1_transpose ==
  euler angles : Inport
  Constant : Constant  Value=zeros(3)
  Constant{1,4,6,8} (4 alike) : Constant  Value=zeros(3,1)
  Constant{10,12,21,25} (4 alike) : Constant  Value=zeros(3,6)
  Constant{11,17,19,23} (4 alike) : Constant  Value=zeros(2,6)
  Constant13 : Constant  Value=zeros(4,1)
  Constant14 : Constant  Value=0
  Constant15 : Constant  Value=zeros(4,1)
  Constant16 : Constant  Value=0
  Constant18 : Constant  Value=zeros(4,6)
  Constant2 : Constant  Value=0
  Constant{20,22,24,26} (4 alike) : Constant  Value=zeros(5,1)
  Constant{3,5,7,9} (4 alike) : Constant  Value=zeros(2,1)
  Create 3x3 Matrix : sharedutil/Create 3x3 Matrix  aMode=aMode
  Demux : Demux  Outputs=3
  Gain{,1..8} (9 alike) : Gain  Gain=-1
  Matrix Concatenate : Concatenate  Mode=Multidimensional array  ConcatenateDimension=2
  Matrix Concatenate{1,3..5,12,14} (6 alike) : Concatenate  NumInputs=3  Mode=Multidimensional array
  Matrix Concatenate{2,6..11,13,15..31} (25 alike) : Concatenate  Mode=Multidimensional array
  Transpose{,1..9} (10 alike) : Math  Operator=transpose  SaturateOnIntegerOverflow=on
  "\\xi_{D2D1C1}" : Outport
  wires:
  euler angles/1 -> Demux/1
  Demux/1 -> [p4], Gain/1, Create 3x3 Matrix/6  "p"
  Gain/1 -> Create 3x3 Matrix/8
  Demux/2 -> [q_4], Create 3x3 Matrix/7, Gain1/1  "q"
  Gain1/1 -> Create 3x3 Matrix/3
  Demux/3 -> Gain2/1, Create 3x3 Matrix/2, [r4]  "r"
  Gain2/1 -> Create 3x3 Matrix/4
  Create 3x3 Matrix/1 -> Gain3/1
  Constant/1 -> Matrix Concatenate/2
  Matrix Concatenate/1 -> Matrix Concatenate2/1
  Constant2/1 -> Create 3x3 Matrix/9, Create 3x3 Matrix/5, Create 3x3 Matrix/1
  Gain3/1 -> Matrix Concatenate/1
  Constant1/1 -> Matrix Concatenate1/1
  Constant3/1 -> Matrix Concatenate1/3
  Gain4/1 -> Matrix Concatenate1/2
  Matrix Concatenate1/1 -> Transpose/1
  Gain5/1 -> Matrix Concatenate3/2
  Constant5/1 -> Matrix Concatenate3/3
  Constant4/1 -> Matrix Concatenate3/1
  Constant7/1 -> Matrix Concatenate4/3
  Constant6/1 -> Matrix Concatenate4/1
  Constant9/1 -> Matrix Concatenate5/3
  Constant8/1 -> Matrix Concatenate5/1
  [q_4] -> Gain4/1
  [r4] -> Gain5/1
  [p4] -> Matrix Concatenate4/2
  [q_4] -> Matrix Concatenate5/2
  Matrix Concatenate2/1 -> Matrix Concatenate6/1
  Constant10/1 -> Matrix Concatenate6/2
  Matrix Concatenate6/1 -> Matrix Concatenate7/1
  Matrix Concatenate3/1 -> Transpose1/1
  Matrix Concatenate7/1 -> Matrix Concatenate8/1
  Matrix Concatenate8/1 -> Matrix Concatenate9/1
  Constant11/1 -> Matrix Concatenate8/2
  Matrix Concatenate4/1 -> Transpose2/1
  Matrix Concatenate9/1 -> Matrix Concatenate10/1
  Constant12/1 -> Matrix Concatenate10/2
  Matrix Concatenate10/1 -> Matrix Concatenate11/1
  Matrix Concatenate5/1 -> Transpose3/1
  Constant13/1 -> Matrix Concatenate12/1
  Constant14/1 -> Matrix Concatenate12/3
  [r4] -> Matrix Concatenate12/2
  Matrix Concatenate12/1 -> Transpose4/1
  Matrix Concatenate11/1 -> Matrix Concatenate13/1
  Constant16/1 -> Matrix Concatenate14/3
  [p4] -> Gain6/1
  Constant15/1 -> Matrix Concatenate14/1
  Gain6/1 -> Matrix Concatenate14/2
  Matrix Concatenate13/1 -> Matrix Concatenate15/1
  Constant17/1 -> Matrix Concatenate15/2
  Matrix Concatenate15/1 -> Matrix Concatenate16/1
  Matrix Concatenate14/1 -> Transpose5/1
  Matrix Concatenate16/1 -> Matrix Concatenate17/1
  Constant18/1 -> Matrix Concatenate17/2
  Matrix Concatenate17/1 -> Matrix Concatenate18/1
  Matrix Concatenate18/1 -> Matrix Concatenate19/1
  Constant19/1 -> Matrix Concatenate19/2
  Matrix Concatenate19/1 -> Matrix Concatenate20/1
  Constant20/1 -> Matrix Concatenate21/1
  Gain7/1 -> Matrix Concatenate21/2
  [q_4] -> Gain7/1
  Matrix Concatenate21/1 -> Transpose6/1
  Matrix Concatenate20/1 -> Matrix Concatenate22/1
  Matrix Concatenate22/1 -> Matrix Concatenate23/1
  Constant21/1 -> Matrix Concatenate23/2
  Matrix Concatenate23/1 -> Matrix Concatenate24/1
  Gain8/1 -> Matrix Concatenate25/2
  Constant22/1 -> Matrix Concatenate25/1
  [r4] -> Gain8/1
  Matrix Concatenate25/1 -> Transpose7/1
  Matrix Concatenate24/1 -> Matrix Concatenate26/1
  Constant23/1 -> Matrix Concatenate26/2
  Matrix Concatenate26/1 -> Matrix Concatenate27/1
  Matrix Concatenate28/1 -> Transpose8/1
  [p4] -> Matrix Concatenate28/2
  Constant24/1 -> Matrix Concatenate28/1
  Matrix Concatenate27/1 -> Matrix Concatenate29/1
  Constant25/1 -> Matrix Concatenate29/2
  Matrix Concatenate29/1 -> Matrix Concatenate30/1
  Constant26/1 -> Matrix Concatenate31/1
  [q_4] -> Matrix Concatenate31/2
  Matrix Concatenate31/1 -> Transpose9/1
  Matrix Concatenate30/1 -> "\\xi_{D2D1C1}"/1
  Transpose/1 -> Matrix Concatenate2/2
  Transpose1/1 -> Matrix Concatenate7/2
  Transpose2/1 -> Matrix Concatenate9/2
  Transpose3/1 -> Matrix Concatenate11/2
  Transpose4/1 -> Matrix Concatenate18/2, Matrix Concatenate13/2
  Transpose5/1 -> Matrix Concatenate16/2, Matrix Concatenate20/2
  Transpose6/1 -> Matrix Concatenate22/2
  Transpose7/1 -> Matrix Concatenate24/2
  Transpose8/1 -> Matrix Concatenate27/2
  Transpose9/1 -> Matrix Concatenate30/2

== system UAV_sync_unknown_sim/Node 4/Node 2/eps_c1_transpose ==
  euler angles : Inport
  Constant : Constant  Value=zeros(3)
  Constant1 : Constant  Value=zeros(6,1)
  Constant{2..3,6..7} (4 alike) : Constant  Value=0
  Constant4 : Constant  Value=zeros(3)
  Constant5 : Constant  Value=zeros(6,1)
  Constant8 : Constant  Value=zeros(3)
  Constant9 : Constant  Value=zeros(6,1)
  Create 3x3 Matrix{,1..3} (4 alike) : sharedutil/Create 3x3 Matrix  aMode=aMode
  Demux : Demux  Outputs=3
  Gain{,1..7} (8 alike) : Gain  Gain=-1
  Matrix Concatenate{,2,5..6} (4 alike) : Concatenate  Mode=Multidimensional array
  Matrix Concatenate{1,3..4,7..9} (6 alike) : Concatenate  Mode=Multidimensional array  ConcatenateDimension=2
  eps_c : Outport
  wires:
  euler angles/1 -> Demux/1
  Demux/1 -> Gain6/1, Create 3x3 Matrix3/2, Gain/1, Create 3x3 Matrix/6, Create 3x3 Matrix1/7, Gain3/1  "p"
  Gain/1 -> Create 3x3 Matrix/8
  Demux/2 -> Create 3x3 Matrix2/1, Gain4/1, Create 3x3 Matrix/7, Gain1/1  "q"
  Gain1/1 -> Create 3x3 Matrix/3
  Demux/3 -> Gain7/1, Create 3x3 Matrix3/6, Create 3x3 Matrix2/5, Gain5/1, Gain2/1, Create 3x3 Matrix/2  "r"
  Gain2/1 -> Create 3x3 Matrix/4
  Create 3x3 Matrix/1 -> Matrix Concatenate/1
  Constant/1 -> Matrix Concatenate/2
  Matrix Concatenate/1 -> Matrix Concatenate1/1
  Constant1/1 -> Matrix Concatenate1/2
  Constant2/1 -> Create 3x3 Matrix/9, Create 3x3 Matrix/5, Create 3x3 Matrix/1
  Constant3/1 -> Create 3x3 Matrix1/8, Create 3x3 Matrix1/6, Create 3x3 Matrix1/4, Create 3x3 Matrix1/3, Create 3x3 Matrix1/2, Create 3x3 Matrix1/1
  Gain3/1 -> Create 3x3 Matrix1/5
  Gain4/1 -> Create 3x3 Matrix1/9
  Create 3x3 Matrix1/1 -> Matrix Concatenate2/2
  Constant4/1 -> Matrix Concatenate2/1
  Matrix Concatenate1/1 -> Matrix Concatenate3/1
  Matrix Concatenate2/1 -> Matrix Concatenate3/2
  Matrix Concatenate3/1 -> Matrix Concatenate4/1
  Constant5/1 -> Matrix Concatenate4/2
  Gain5/1 -> Create 3x3 Matrix2/3
  Constant6/1 -> Create 3x3 Matrix2/9, Create 3x3 Matrix2/8, Create 3x3 Matrix2/7, Create 3x3 Matrix2/6, Create 3x3 Matrix2/4, Create 3x3 Matrix2/2
  Gain6/1 -> Create 3x3 Matrix3/4
  Gain7/1 -> Create 3x3 Matrix3/8
  Constant7/1 -> Create 3x3 Matrix3/9, Create 3x3 Matrix3/7, Create 3x3 Matrix3/5, Create 3x3 Matrix3/3, Create 3x3 Matrix3/1
  Create 3x3 Matrix2/1 -> Matrix Concatenate5/2
  Constant8/1 -> Matrix Concatenate6/1, Matrix Concatenate5/1
  Create 3x3 Matrix3/1 -> Matrix Concatenate6/2
  Constant9/1 -> Matrix Concatenate7/2
  Matrix Concatenate5/1 -> Matrix Concatenate7/1
  Matrix Concatenate7/1 -> Matrix Concatenate8/1
  Matrix Concatenate6/1 -> Matrix Concatenate8/2
  Matrix Concatenate4/1 -> Matrix Concatenate9/1
  Matrix Concatenate8/1 -> Matrix Concatenate9/2
  Matrix Concatenate9/1 -> eps_c/1

== system UAV_sync_unknown_sim/Node 4/Node 2/eps_g ==
  euler angles : Inport
  Cos : Trigonometry  Operator=cos
  Cos1 : Trigonometry  Operator=cos
  Demux : Demux  Outputs=3
  Gain : Gain  Gain=G
  Gain1 : Gain  Gain=G
  Gain2 : Gain  Gain=G
  Gain3 : Gain  Gain=-1
  Gain4 : Gain  Gain=-1
  Multiply : Product
  Multiply1 : Product
  Mux : Mux  Inputs=6
  Sin : Trigonometry
  Sin1 : Trigonometry
  Sin2 : Trigonometry  Operator=cos
  Terminator : Terminator
  Zero : Constant  Value=0  OutDataTypeStr=Inherit: Inherit via back propagation
  eps_g : Outport
  wires:
  euler angles/1 -> Demux/1
  Sin/1 -> Gain/1
  Cos/1 -> Multiply/1
  Sin1/1 -> Multiply/2
  Multiply/1 -> Gain1/1
  Cos1/1 -> Multiply1/1
  Sin2/1 -> Multiply1/2
  Multiply1/1 -> Gain2/1
  Gain/1 -> Mux/1
  Gain1/1 -> Gain3/1
  Gain2/1 -> Gain4/1
  Zero/1 -> Mux/6, Mux/4, Mux/5
  Mux/1 -> eps_g/1
  Gain3/1 -> Mux/2
  Gain4/1 -> Mux/3
  Demux/1 -> Cos1/1, Sin1/1
  Demux/2 -> Sin2/1, Cos/1, Sin/1
  Demux/3 -> Terminator/1

== system UAV_sync_unknown_sim/Node 0/Node 0/Inverse Dynamics Control/Inverse Dynamic 1 ==
  References : Inport
  Aircraft Data : Inport  Port=2
  Add2 : Sum  Inputs=-+
  Bus Selector2 : BusSelector  OutputSignals=xyh_body,Euler angles (rad),Velocity (body),Angular rates (body)
  Bus Selector3 : BusSelector  OutputSignals=xddot_ref_final,yddot_ref_final,hddot_ref_final,phiddot_ref_final,thetaddot_ref_final,psiddot_ref_final
  Constant10 : Constant  Value=D0
  Gain3 : Gain  Gain=-1
  Inner Controller : Subsystem
  Mux1 : Mux  Inputs=6
  Mux5 : Mux  Inputs=6
  Product1 : Product  Multiplication=Matrix(*)
  Subsystem : Subsystem
  D_qddot : Outport
  wires:
  Aircraft Data/1 -> Bus Selector2/1
  Subsystem/4(e_phi) -> Inner Controller/4(e_phi)
  Subsystem/3(e_z) -> Inner Controller/3(e_z)
  Subsystem/5(e_theta) -> Inner Controller/5(e_theta)
  Bus Selector2/1 -> Subsystem/1(<xyh>)  "<xyh_body>"
  Subsystem/2(e_y) -> Inner Controller/2(e_y)
  Mux5/1 -> Add2/1
  Subsystem/6(e_psi) -> Inner Controller/6(e_psi)
  Product1/1 -> D_qddot/1
  Add2/1 -> Product1/2
  Inner Controller/3(act3) -> Gain3/1
  Constant10/1 -> Product1/1
  Mux1/1 -> Add2/2
  Bus Selector2/2 -> Subsystem/2(<Euler angles (rad)>)  "<Euler angles (rad)>"
  Inner Controller/1(act1) -> Mux5/1
  Subsystem/1(e_x) -> Inner Controller/1(e_x)
  Inner Controller/5(act5) -> Mux5/5
  Inner Controller/6(act6) -> Mux5/6
  Inner Controller/4(act4) -> Mux5/4
  Bus Selector2/3 -> Subsystem/3(velocity)  "<Velocity (body)>"
  Subsystem/7(e_xdot) -> Inner Controller/7(e_xdot)
  Bus Selector2/4 -> Subsystem/4(angular_rate)  "<Angular rates (body)>"
  Subsystem/8(e_zdot) -> Inner Controller/8(e_zdot)
  Subsystem/9(e_phidot) -> Inner Controller/9(e_phidot)
  Subsystem/10(e_thetadot) -> Inner Controller/10(e_thetadot)
  Subsystem/11(e_psidot) -> Inner Controller/11(e_psidot)
  Subsystem/12(e_ydot) -> Inner Controller/12(e_ydot)
  Inner Controller/2(act2) -> Mux5/2
  Bus Selector3/1 -> Mux1/1  "<xddot_ref_final>"
  Bus Selector3/2 -> Mux1/2  "<yddot_ref_final>"
  Bus Selector3/3 -> Mux1/3  "<hddot_ref_final>"
  Bus Selector3/4 -> Mux1/4  "<phiddot_ref_final>"
  Bus Selector3/5 -> Mux1/5  "<thetaddot_ref_final>"
  Bus Selector3/6 -> Mux1/6  "<psiddot_ref_final>"
  References/1 -> Subsystem/5(Reference), Bus Selector3/1
  Gain3/1 -> Mux5/3

== system UAV_sync_unknown_sim/Node 0/Node 0/Inverse Dynamics Control/Inverse Dynamic 2 ==
  Aricraft Data : Inport
  Bus Selector1 : BusSelector  OutputSignals=Velocity (body),Angular rates (body)
  Constant1 : Constant  Value=I0(3)
  Constant2 : Constant  Value=I0(1)
  Constant3 : Constant  Value=M0
  Constant4 : Constant  Value=I0(5)
  Constant5 : Constant  Value=I0(9)
  Constant6 : Constant  Value=[0 0 0;0 0 0;0 0 0]
  Constant7 : Constant  Value=0
  Matrix Concatenate : Concatenate  Mode=Multidimensional array  ConcatenateDimension=2
  Matrix Concatenate1 : Concatenate  Mode=Multidimensional array  ConcatenateDimension=2
  Matrix Concatenate2 : Concatenate  Mode=Multidimensional array
  Mux1 : Mux  Inputs=2
  Product2 : Product  Multiplication=Matrix(*)
  Rot_Matrix [3x3] : Subsystem
  Trans_Matrix [3x3] : Subsystem
  p : Fcn  Expr=u(1)
  q : Fcn  Expr=u(2)
  r : Fcn  Expr=u(3)
  C_qdot : Outport
  wires:
  Aricraft Data/1 -> Bus Selector1/1
  Matrix Concatenate/1 -> Matrix Concatenate2/1
  Matrix Concatenate1/1 -> Matrix Concatenate2/2
  Rot_Matrix [3x3]/1(Out1) -> Matrix Concatenate1/2
  Constant7/1 -> Trans_Matrix [3x3]/4(zero), Rot_Matrix [3x3]/4(Zero)
  Constant3/1 -> Trans_Matrix [3x3]/5(M)
  r/1 -> Rot_Matrix [3x3]/3(r), Trans_Matrix [3x3]/3(r)
  Constant2/1 -> Rot_Matrix [3x3]/5(I1)
  Trans_Matrix [3x3]/1(Out1) -> Matrix Concatenate/1
  Bus Selector1/1 -> Mux1/1  "<Velocity (body)>"
  Constant4/1 -> Rot_Matrix [3x3]/6(I5)
  Matrix Concatenate2/1 -> Product2/1
  Bus Selector1/2 -> Mux1/2, p/1, q/1, r/1  "<Angular rates (body)>"
  Constant5/1 -> Rot_Matrix [3x3]/7(I9)
  Constant6/1 -> Matrix Concatenate/2, Matrix Concatenate1/1
  q/1 -> Rot_Matrix [3x3]/2(q), Trans_Matrix [3x3]/2(q)
  p/1 -> Rot_Matrix [3x3]/1(p), Trans_Matrix [3x3]/1(p)
  Product2/1 -> C_qdot/1
  Mux1/1 -> Product2/2
  Constant1/1 -> Rot_Matrix [3x3]/8(I3_I7)

== system UAV_sync_unknown_sim/Node 0/VF Approach/AUTOPILOT/Fly-by-wire inputs ==
  note: Put here your custom inputs
  Thr in : Inport
  Pitch in : Inport  Port=2
  . : Inport  Port=3
  Roll in : Inport  Port=4
  Constant : Constant  Commented=on  Value=0
  Dummy port : Terminator
  From Workspace : FromWorkspace  Commented=on  VariableName=LogData.RCIN.Throttle_IN  SampleTime=0.001
  From Workspace1 : FromWorkspace  Commented=on  VariableName=LogData.RCIN.Pitch_IN  SampleTime=0.001
  From Workspace2 : FromWorkspace  Commented=on  VariableName=LogData.RCIN.Roll_IN  SampleTime=0.001
  Manual Switch1 : ManualSwitch  CurrentSetting=0
  Manual Switch2 : ManualSwitch
  Manual Switch3 : ManualSwitch
  Manual Switch4 : ManualSwitch
  Thr out : Outport
  Pitch out : Outport  Port=2
  Roll out : Outport  Port=3
  tag scope: PitchDem=scoped, RollDem=scoped, ThrottleDem=scoped
  wires:
  Manual Switch3/1 -> Pitch out/1
  Manual Switch1/1 -> Thr out/1
  Pitch in/1 -> [PitchDem], Manual Switch3/1
  From Workspace/1 -> Manual Switch1/1
  Manual Switch2/1 -> [RollDem], Roll out/1
  Roll in/1 -> Manual Switch2/1
  From Workspace1/1 -> Manual Switch3/2
  Thr in/1 -> [ThrottleDem], Manual Switch1/2
  Constant/1 -> Manual Switch4/2
  From Workspace2/1 -> Manual Switch4/1
  Manual Switch4/1 -> Manual Switch2/2
  ./1 -> Dummy port/1

== system UAV_sync_unknown_sim/Node 0/VF Approach/AUTOPILOT/Low-level Controllers ==
  ThrottIn : Inport  Unit=%
  Pitch : Inport  Port=2  Unit=deg
  Roll : Inport  Port=3  Unit=deg
  PlantData : Inport  Port=4
  Angle Conversion1 : aerolibconvert2/Angle Conversion  IU=rad  OU=deg
  Angle Conversion2 : aerolibconvert2/Angle Conversion  IU=rad  OU=deg
  Angular Velocity Conversion : aerolibconvert2/Angular Velocity Conversion  IU=rad/s  OU=deg/s
      settings: SourceProductName=Aerospace Blockset
  Angular Velocity Conversion1 : aerolibconvert2/Angular Velocity Conversion  IU=rad/s  OU=deg/s
      settings: SourceProductName=Aerospace Blockset
  Bus Selector : BusSelector  OutputSignals=Euler angles (rad)
  Bus Selector1 : BusSelector  OutputSignals=Angular rates (body) (rad/s)
  Bus Selector2 : BusSelector  OutputSignals=Euler angles (rad)
  Bus Selector3 : BusSelector  OutputSignals=Angular rates (body) (rad/s)
  Bus Selector5 : BusSelector  OutputSignals=Angular rates (body) (rad/s)
  Bus Selector6 : BusSelector  OutputSignals=Euler angles (rad)
  Bus Selector7 : BusSelector  OutputSignals=Accelerations (body/body)
  Get scaling factor : Subsystem
  Pitch controller : Subsystem
  Roll controller : Subsystem
  Side-slip angle controller : Subsystem
  ThrottOut : Outport  Unit=%
  AilDemand : Outport  Port=2  Unit=deg
  ElevDemand : Outport  Port=3  Unit=deg
  RuddDemand : Outport  Port=4  Unit=deg
  wires:
  Bus Selector/1 -> Angle Conversion1/1  "<Euler angles (rad)>"
  Roll controller/1(AilDemand) -> [AilDem], AilDemand/1
  Bus Selector1/1 -> Angular Velocity Conversion1/1  "<Angular rates (body) (rad/s)>"
  Bus Selector2/1 -> Angle Conversion2/1  "<Euler angles (rad)>"
  Bus Selector3/1 -> Angular Velocity Conversion/1  "<Angular rates (body) (rad/s)>"
  Pitch controller/1(ElevDemand) -> ElevDemand/1
  Get scaling factor/1(Scaler) -> Roll controller/4(Scaler), Side-slip angle controller/4(Scaler), Pitch controller/4(Scaler)
  Bus Selector7/1 -> Side-slip angle controller/3(accel_y)  "<Accelerations (body/body)>"
  Bus Selector6/1 -> Side-slip angle controller/2("Euler angles ")  "<Euler angles (rad)>"
  Bus Selector5/1 -> Side-slip angle controller/1(Yaw_rate)  "<Angular rates (body) (rad/s)>"
  [PlantData] -> Bus Selector1/1, Bus Selector2/1, Bus Selector3/1, Bus Selector5/1, Bus Selector6/1, Bus Selector7/1, Bus Selector/1
  Pitch/1 -> [PitchRef]
  PlantData/1 -> [PlantData]
  ThrottIn/1 -> ThrottOut/1
  Angle Conversion2/1 -> Pitch controller/2(EulerAngles)
  Angular Velocity Conversion/1 -> Pitch controller/3(AngularRates)
  Angle Conversion1/1 -> Roll controller/2(Euler angles)
  Angular Velocity Conversion1/1 -> Roll controller/3(AngularRates)
  Roll/1 -> [RollRef]
  [PitchRef] -> Pitch controller/1(PitchReference)
  [RollRef] -> Roll controller/1(RollReference)
  [AilDem] -> Side-slip angle controller/5(AilDemand)
  Side-slip angle controller/1(RudderDemand) -> RuddDemand/1
